simulink model "CH22_3F"  (Simulink 10.1)
settings: Solver=ode45  StartTime=0.0  StopTime=2000  RelTol=1e-3  EnableMultiTasking=on
libraries: commfilt2 x2, commrandsrc2 x2, commutil2 x2
settings Model: Creator=my2  LastModifiedBy=IT
settings DataIOCC: LimitDataPoints=on  SignalLoggingSaveFormat=ModelDataLogs
settings DebuggingCC: SolverPrmCheckMsg=warning  FcnCallInpInsideContextMsg=warning

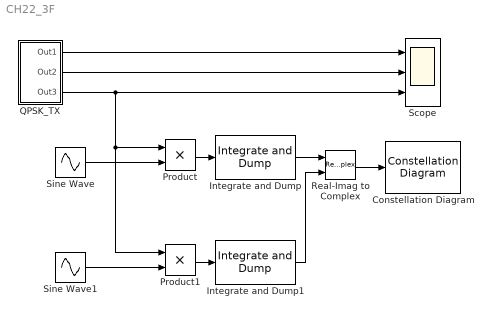
== system CH22_3F ==
  Constellation Diagram : ConstellationDiagram  Tag=ScatterPlot
  Integrate and Dump : commfilt2/Integrate and Dump  obssamples=8  offsetsamples=0  nodump=off  roundingMode=Floor  overflowMode=off  outputDataTypeStr=Inherit: Same as accumulator  outputLastDataTypeStr=Inherit: Same as accumulator
  Integrate and Dump1 : commfilt2/Integrate and Dump  obssamples=8  offsetsamples=0  nodump=off  roundingMode=Floor  overflowMode=off  outputDataTypeStr=Inherit: Same as accumulator  outputLastDataTypeStr=Inherit: Same as accumulator
  Product : Product
  Product1 : Product
  QPSK_TX : Subsystem
  Real-Imag to Complex : RealImagToComplex
  Scope : Scope  NumInputPorts=3
  Sine Wave : Sin  SampleTime=1/256
  Sine Wave1 : Sin  SampleTime=1/256
  wires:
  QPSK_TX/1(Out1) -> Scope/1
  QPSK_TX/2(Out2) -> Scope/2
  Sine Wave/1 -> Product/2
  Product/1 -> Integrate and Dump/1
  QPSK_TX/3(Out3) -> Product/1, Product1/1, Scope/3
  Sine Wave1/1 -> Product1/2
  Product1/1 -> Integrate and Dump1/1
  Integrate and Dump/1 -> Real-Imag to Complex/1
  Integrate and Dump1/1 -> Real-Imag to Complex/2
  Real-Imag to Complex/1 -> Constellation Diagram/1

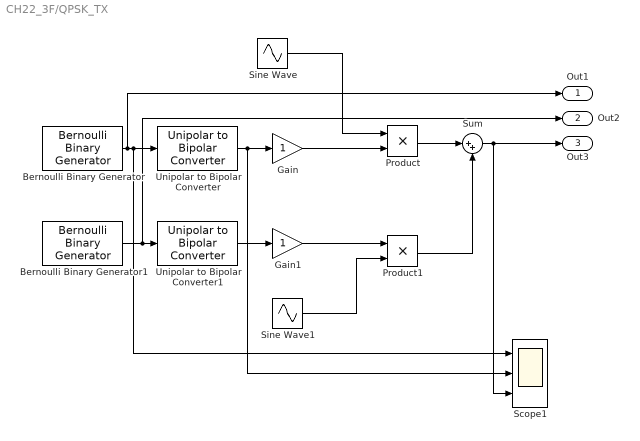
== system CH22_3F/QPSK_TX ==
  Bernoulli Binary Generator : commrandsrc2/Bernoulli Binary Generator  P=0.5  seed=20301181  Ts=1  frameBased=off  sampPerFrame=1  orient=off  outDataType=boolean
      settings: SourceProductBaseCode=CM
  Bernoulli Binary Generator1 : commrandsrc2/Bernoulli Binary Generator  P=0.5  seed=7  Ts=1  frameBased=off  sampPerFrame=1  orient=off  outDataType=boolean
      settings: SourceProductBaseCode=CM
  Gain : Gain
  Gain1 : Gain
  Product : Product
  Product1 : Product
  Scope1 : Scope  NumInputPorts=3
  Sine Wave : Sin  SampleTime=1/256
  Sine Wave1 : Sin  SampleTime=1/256
  Sum : Sum  Inputs=|++
  Unipolar to Bipolar Converter : commutil2/Unipolar to Bipolar Converter  M=2  polarity=Positive  dataType=Inherit via internal rule
  Unipolar to Bipolar Converter1 : commutil2/Unipolar to Bipolar Converter  M=2  polarity=Positive  dataType=Inherit via internal rule
  Out1 : Outport
  Out2 : Outport  Port=2
  Out3 : Outport  Port=3
  wires:
  Sum/1 -> Scope1/3, Out3/1
  Unipolar to Bipolar Converter/1 -> Scope1/2, Gain/1
  Sine Wave1/1 -> Product1/2
  Gain1/1 -> Product1/1
  Sine Wave/1 -> Product/1
  Bernoulli Binary Generator/1 -> Out1/1, Scope1/1, Unipolar to Bipolar Converter/1
  Product/1 -> Sum/1
  Product1/1 -> Sum/2
  Unipolar to Bipolar Converter1/1 -> Gain1/1
  Bernoulli Binary Generator1/1 -> Out2/1, Unipolar to Bipolar Converter1/1
  Gain/1 -> Product/2
